simulink model "LDW_mask"  (Simulink 7.8)
settings: Solver=FixedStepDiscrete  StartTime=0.0  StopTime=10.0  FixedStep=1/100  RelTol=1e-3
undefined symbols (not defined in the file or in its folder): High, num_targets, slselsubs
libraries: simulink x35, dspmtrx3 x13, visiontextngfix x9, dspsigops x6, simulink_extras x4, visiontransforms x4, dspstat3 x4, dspswit3 x3, dspadpt3 x3, dspindex x2, visionconversions x2, visionstatistics x2
(part 2 of 3)

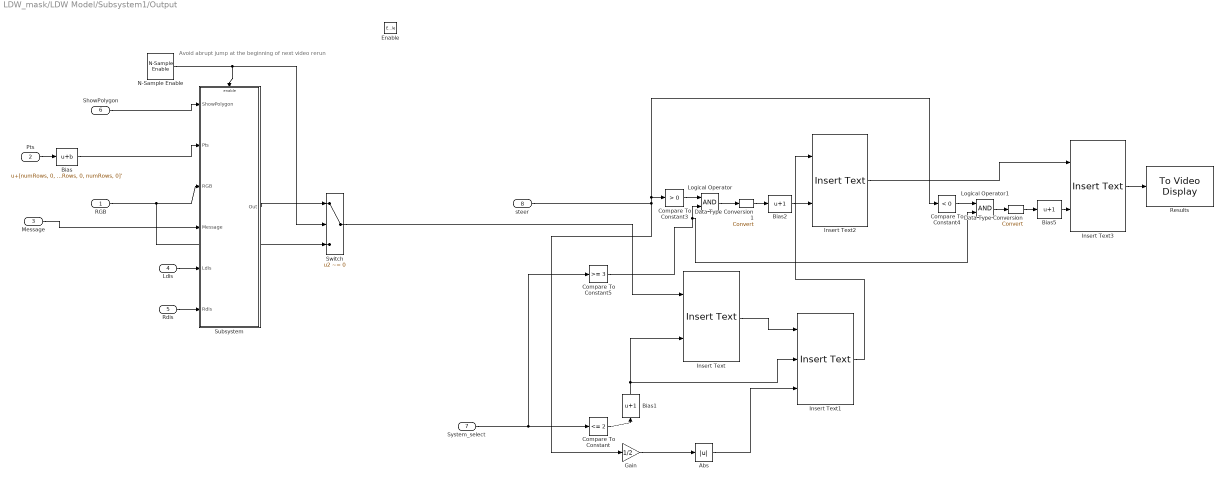
== system LDW_mask/LDW Model/Subsystem1/Output ==
  note: Avoid abrupt jump at the beginning of next video rerun
  RGB : Inport
  Pts : Inport  Port=2
  Message : Inport  Port=3
  Ldis : Inport  Port=4
  Rdis : Inport  Port=5
  ShowPolygon : Inport  Port=6
  System_select : Inport  Port=7
  steer : Inport  Port=8
  Enable : EnablePort
  Abs : Abs
  Bias : Bias  Bias=[numRows, 0, numRows, 0; numRows, 0, numRows, 0]'
  Bias1 : Bias  Bias=1
  Bias2 : Bias  Bias=1
  Bias5 : Bias  Bias=1
  Compare To Constant : simulink/Logic and Bit Operations/Compare To Constant  relop=<=  const=2  OutDataTypeStr=uint8
  Compare To Constant3 : simulink/Logic and Bit Operations/Compare To Constant  relop=>  const=0  OutDataTypeStr=uint8
  Compare To Constant4 : simulink/Logic and Bit Operations/Compare To Constant  relop=<  const=0  OutDataTypeStr=uint8
  Compare To Constant5 : simulink/Logic and Bit Operations/Compare To Constant  relop=>=  const=3  OutDataTypeStr=uint8
  Data Type Conversion : DataTypeConversion
  Data Type Conversion1 : DataTypeConversion
  Gain : Gain  Gain=1/2  OutDataTypeStr=Inherit: Inherit via back propagation
  Insert Text : visiontextngfix/Insert Text  inputType=Obsolete  theText={'Steer:' , ''}  fontFace=LucidaTypewriterBold  dummyVar1=0  blockFontSize=14  antiAliased=on  getTextLocFrom=Specify via dialog  textLoc=[240 10]  getTextColorFrom=Specify via dialog  textColor=[210/255 105/255 30/255]  getTextIntensityFrom=Specify via dialog  textIntensity=0  getTextOpacityFrom=Specify via dialog  textOpacity=1  dummyVar2=0  dummyVar3=0  dummyVar4=0  imagePorts=One multidimensional signal  isInputTransposed=off
  Insert Text1 : visiontextngfix/Insert Text  inputType=Obsolete  theText={[' %6.1f%%'] , ''}  fontFace=LucidaTypewriterBold  dummyVar1=0  blockFontSize=14  antiAliased=on  getTextLocFrom=Specify via dialog  textLoc=[220 25]  getTextColorFrom=Specify via dialog  textColor=[210/255 105/255 30/255]  getTextIntensityFrom=Specify via dialog  textIntensity=0  getTextOpacityFrom=Specify via dialog  textOpacity=1  dummyVar2=0  dummyVar3=0  dummyVar4=0  imagePorts=One multidimensional signal  isInputTransposed=off
  Insert Text2 : visiontextngfix/Insert Text  inputType=Obsolete  theText={'','Left' }  fontFace=LucidaTypewriterBold  dummyVar1=0  blockFontSize=14  antiAliased=on  getTextLocFrom=Specify via dialog  textLoc=[170 10]  getTextColorFrom=Specify via dialog  textColor=[210/255 105/255 30/255]  getTextIntensityFrom=Specify via dialog  textIntensity=0  getTextOpacityFrom=Specify via dialog  textOpacity=1  dummyVar2=0  dummyVar3=0  dummyVar4=0  imagePorts=One multidimensional signal  isInputTransposed=off
  Insert Text3 : visiontextngfix/Insert Text  inputType=Obsolete  theText={'','Right' }  fontFace=LucidaTypewriterBold  dummyVar1=0  blockFontSize=14  antiAliased=on  getTextLocFrom=Specify via dialog  textLoc=[315 10]  getTextColorFrom=Specify via dialog  textColor=[210/255 105/255 30/255]  getTextIntensityFrom=Specify via dialog  textIntensity=0  getTextOpacityFrom=Specify via dialog  textOpacity=1  dummyVar2=0  dummyVar3=0  dummyVar4=0  imagePorts=One multidimensional signal  isInputTransposed=off
  Logical Operator : Logic  AllPortsSameDT=off  OutDataTypeStr=boolean
  Logical Operator1 : Logic  AllPortsSameDT=off  OutDataTypeStr=boolean
  N-Sample Enable : dspswit3/N-Sample Enable  N=8  ActiveLevel=High (1)  reset=off  TriggerType=Non-zero sample  Ts=vfq  DataType=Logical
  Results : visionsinks/To Video Display  inputType=Obsolete  imagePorts=One multidimensional signal  OutputDevice=On-screen video monitor  fullScreen=off  videoWindowX=19  videoWindowY=34  saveWindowSize=off  videoWindowWidth=500  videoWindowHeight=375  dataOrg=Column-major  openAtMdlStart=on  isWindowOpen=on  inputColorFormat=RGB
  Subsystem : Subsystem
  Switch : Switch  Criteria=u2 ~= 0
  wires:
  Pts/1 -> Bias/1
  Message/1 -> Subsystem/4(Message)
  Bias/1 -> Subsystem/2(Pts)
  Subsystem/1(Out) -> Switch/1
  ShowPolygon/1 -> Subsystem/1(ShowPolygon)
  RGB/1 -> Subsystem/3(RGB), Switch/3
  N-Sample Enable/1 -> Subsystem/Enable, Switch/2
  Switch/1 -> Insert Text/1
  Ldis/1 -> Subsystem/5(Ldis)
  Rdis/1 -> Subsystem/6(Rdis)
  System_select/1 -> Compare To Constant/1, Compare To Constant5/1
  Insert Text/1 -> Insert Text1/1
  Compare To Constant/1 -> Bias1/1
  Gain/1 -> Abs/1
  Logical Operator1/1 -> Data Type Conversion/1
  steer/1 -> Compare To Constant4/1, Compare To Constant3/1, Gain/1
  Compare To Constant3/1 -> Logical Operator/1
  Compare To Constant4/1 -> Logical Operator1/1
  Logical Operator/1 -> Data Type Conversion1/1
  Insert Text2/1 -> Insert Text3/1
  Insert Text1/1 -> Insert Text2/1
  Compare To Constant5/1 -> Logical Operator1/2, Logical Operator/2
  Abs/1 -> Insert Text1/3
  Insert Text3/1 -> Results/1
  Data Type Conversion/1 -> Bias5/1
  Bias5/1 -> Insert Text3/2
  Data Type Conversion1/1 -> Bias2/1
  Bias2/1 -> Insert Text2/2
  Bias1/1 -> Insert Text/2, Insert Text1/2

== system LDW_mask/LDW Model/Subsystem1/ind_light ==
  ind_flag : Inport
  ldw_message : Inport  Port=2
  Compare To Constant : simulink/Logic and Bit Operations/Compare To Constant  relop===  const=2  OutDataTypeStr=uint8
  Compare To Constant1 : Logic  AllPortsSameDT=off  OutDataTypeStr=boolean
  Compare To Constant2 : Logic  AllPortsSameDT=off  OutDataTypeStr=boolean
  Compare To Constant3 : Logic  Operator=NOT  AllPortsSameDT=off  OutDataTypeStr=boolean
  Constant : Constant  Value=0
  Constant1 : Constant  Value=0
  Pulse Generator : DiscretePulseGenerator  Period=76  PulseWidth=76/2  SampleTime=Ts_ind
  Pulse Generator1 : DiscretePulseGenerator  Period=76  PulseWidth=76/2  SampleTime=Ts_ind
  Rate Transition : RateTransition  OutPortSampleTimeOpt=Inherit
  Rate Transition1 : RateTransition  OutPortSampleTimeOpt=Inherit
  Switch : Switch  Criteria=u2 > Threshold  Threshold=0.5
  Switch1 : Switch  Criteria=u2 > Threshold  Threshold=0.5
  no : simulink/Logic and Bit Operations/Compare To Constant  relop===  const=0  OutDataTypeStr=uint8
  light_left : Outport
  light_right : Outport  Port=2
  wires:
  Pulse Generator/1 -> Switch/1
  Switch/1 -> light_left/1
  Constant/1 -> Switch/3
  Pulse Generator1/1 -> Switch1/1
  Constant1/1 -> Switch1/3
  Switch1/1 -> light_right/1
  ldw_message/1 -> Compare To Constant/1, no/1
  Compare To Constant/1 -> Compare To Constant2/2
  Compare To Constant2/1 -> Rate Transition1/1
  Compare To Constant1/1 -> Rate Transition/1
  no/1 -> Compare To Constant1/1
  Rate Transition/1 -> Switch1/2
  Rate Transition1/1 -> Switch/2
  ind_flag/1 -> Compare To Constant3/1
  Compare To Constant3/1 -> Compare To Constant2/1, Compare To Constant1/2

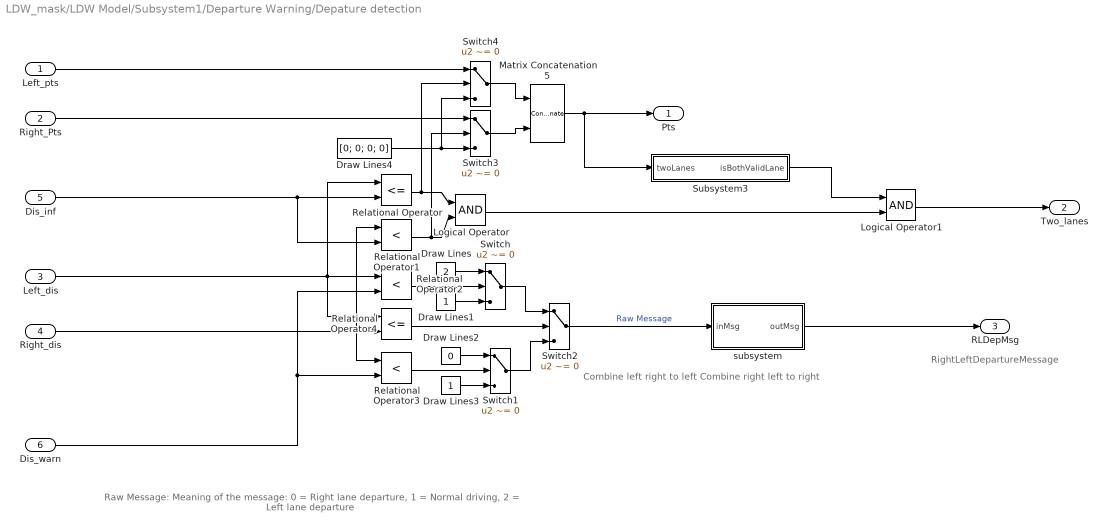
== system LDW_mask/LDW Model/Subsystem1/Departure Warning/Depature detection ==
  note: Raw Message:
      | Meaning of the message: 0 = Right lane departure, 1 = Normal driving, 2 = Left lane departure
  note: RightLeftDepartureMessage
  note: Combine left right to left
      | Combine right left to right
  Left_pts : Inport
  Right_Pts : Inport  Port=2
  Left_dis : Inport  Port=3
  Right_dis : Inport  Port=4
  Dis_inf : Inport  Port=5
  Dis_warn : Inport  Port=6
  Draw Lines : Constant  Value=2  VectorParams1D=off  OutDataTypeStr=int8  SampleTime=cfq
  Draw Lines1 : Constant  VectorParams1D=off  OutDataTypeStr=int8  SampleTime=cfq
  Draw Lines2 : Constant  Value=0  VectorParams1D=off  OutDataTypeStr=int8  SampleTime=cfq
  Draw Lines3 : Constant  VectorParams1D=off  OutDataTypeStr=int8  SampleTime=cfq
  Draw Lines4 : Constant  Value=[0; 0; 0; 0]  VectorParams1D=off  OutDataTypeStr=int32  SampleTime=cfq
  Logical Operator : Logic  AllPortsSameDT=off  OutDataTypeStr=boolean
  Logical Operator1 : Logic  AllPortsSameDT=off  OutDataTypeStr=boolean  SampleTime=cfq
  Matrix Concatenation5 : Concatenate  Mode=Multidimensional array  ConcatenateDimension=2
  Relational Operator : RelationalOperator  Operator=<=  OutDataTypeStr=boolean  ZeroCross=off
  Relational Operator1 : RelationalOperator  Operator=<  OutDataTypeStr=boolean  ZeroCross=off
  Relational Operator2 : RelationalOperator  Operator=<  OutDataTypeStr=boolean  ZeroCross=off
  Relational Operator3 : RelationalOperator  Operator=<  OutDataTypeStr=boolean  ZeroCross=off
  Relational Operator4 : RelationalOperator  Operator=<=  OutDataTypeStr=boolean  ZeroCross=off
  Subsystem3 : Subsystem
  Switch : Switch  Criteria=u2 ~= 0
  Switch1 : Switch  Criteria=u2 ~= 0
  Switch2 : Switch  Criteria=u2 ~= 0
  Switch3 : Switch  Criteria=u2 ~= 0  ZeroCross=off
  Switch4 : Switch  Criteria=u2 ~= 0  ZeroCross=off
  subsystem : Subsystem
  Pts : Outport
  Two_lanes : Outport  Port=2
  RLDepMsg : Outport  Port=3
  wires:
  Relational Operator1/1 -> Logical Operator/2, Switch3/2
  Relational Operator/1 -> Logical Operator/1, Switch4/2
  Switch1/1 -> Switch2/3
  Switch/1 -> Switch2/1
  Relational Operator4/1 -> Switch2/2
  Draw Lines3/1 -> Switch1/3
  Draw Lines2/1 -> Switch1/1
  Draw Lines1/1 -> Switch/3
  Draw Lines/1 -> Switch/1
  Relational Operator3/1 -> Switch1/2
  Relational Operator2/1 -> Switch/2
  Dis_warn/1 -> Relational Operator2/2, Relational Operator3/2
  Left_dis/1 -> Relational Operator2/1, Relational Operator4/1, Relational Operator/1
  Right_dis/1 -> Relational Operator1/1, Relational Operator4/2, Relational Operator3/1
  Dis_inf/1 -> Relational Operator/2, Relational Operator1/2
  Switch3/1 -> Matrix Concatenation5/2
  Switch4/1 -> Matrix Concatenation5/1
  Draw Lines4/1 -> Switch3/3, Switch4/3
  Left_pts/1 -> Switch4/1
  Matrix Concatenation5/1 -> Subsystem3/1(twoLanes), Pts/1
  Right_Pts/1 -> Switch3/1
  Switch2/1 -> subsystem/1(inMsg)  "Raw Message"
  subsystem/1(outMsg) -> RLDepMsg/1
  Subsystem3/1(isBothValidLane) -> Logical Operator1/1
  Logical Operator/1 -> Logical Operator1/2
  Logical Operator1/1 -> Two_lanes/1

== system LDW_mask/LDW Model/Subsystem1/Departure Warning/Depature detection1 ==
  note: Combine left right to left
      | Combine right left to right
  note: RightLeftDepartureMessage
  Left_dis : Inport
  Right_dis : Inport  Port=2
  Dis_LDW_warn : Inport  Port=3
  Enable : EnablePort
  Draw Lines : Constant  Value=2  VectorParams1D=off  OutDataTypeStr=int8  SampleTime=cfq
  Draw Lines1 : Constant  VectorParams1D=off  OutDataTypeStr=int8  SampleTime=cfq
  Draw Lines2 : Constant  Value=0  VectorParams1D=off  OutDataTypeStr=int8  SampleTime=cfq
  Draw Lines3 : Constant  VectorParams1D=off  OutDataTypeStr=int8  SampleTime=cfq
  Relational Operator2 : RelationalOperator  Operator=<  OutDataTypeStr=boolean  ZeroCross=off
  Relational Operator3 : RelationalOperator  Operator=<  OutDataTypeStr=boolean  ZeroCross=off
  Relational Operator4 : RelationalOperator  Operator=<=  OutDataTypeStr=boolean  ZeroCross=off
  Switch : Switch  Criteria=u2 ~= 0
  Switch1 : Switch  Criteria=u2 ~= 0
  Switch2 : Switch  Criteria=u2 ~= 0
  subsystem : Subsystem
  LDW_Asist_flag : Outport
  wires:
  subsystem/1(outMsg) -> LDW_Asist_flag/1
  Switch2/1 -> subsystem/1(inMsg)  "Raw Massage"
  Right_dis/1 -> Relational Operator3/1, Relational Operator4/2
  Left_dis/1 -> Relational Operator4/1, Relational Operator2/1
  Dis_LDW_warn/1 -> Relational Operator3/2, Relational Operator2/2
  Relational Operator2/1 -> Switch/2
  Relational Operator3/1 -> Switch1/2
  Draw Lines/1 -> Switch/1
  Draw Lines1/1 -> Switch/3
  Draw Lines2/1 -> Switch1/1
  Draw Lines3/1 -> Switch1/3
  Relational Operator4/1 -> Switch2/2
  Switch/1 -> Switch2/1
  Switch1/1 -> Switch2/3

== system LDW_mask/LDW Model/Subsystem1/Departure Warning/Find the left and  right lanes from the depository ==
  note: Left and right lanes are identified by their intersection positions with the bottom image boundary.
      | The intersection point of the left lane is to the left of the image bottom boundary center,
      | and is the one closest to the center. By the same way, but to the right, the right lane is defined.
  Count : Inport
  Pts : Inport  Port=2
  Half_width : Inport  Port=3
  Dis_inf : Inport  Port=4
  Compare To Constant2 : simulink/Logic and Bit Operations/Compare To Constant  relop=>=  const=frameFound  OutDataTypeStr=boolean  ZeroCross=off
  For Iterator : ForIterator  ResetStates=reset  IterationLimit=maxLaneNum
  Search for the left and right lanes : Subsystem
  select rho1 : Selector  NumberOfDimensions=2  InputPortWidth=maxLaneNum  IndexOptions=Select all,Index vector (port)  Indices=-1,-1  OutputSizes=1
  select rho5 : Selector  NumberOfDimensions=2  InputPortWidth=maxLaneNum  IndexOptions=Select all,Index vector (port)  Indices=-1,-1  OutputSizes=1
  Left_pts : Outport
  Left_dis : Outport  Port=2
  wires:
  Pts/1 -> select rho5/1
  select rho1/1 -> Compare To Constant2/1
  Half_width/1 -> Search for the left and right lanes/3(Half_width)
  select rho5/1 -> Search for the left and right lanes/2(Pts)
  Compare To Constant2/1 -> Search for the left and right lanes/1(Enable)
  Search for the left and right lanes/1(Left_pts) -> Left_pts/1
  Search for the left and right lanes/2(Left_dis) -> Left_dis/1
  For Iterator/1 -> select rho5/2, select rho1/2
  Count/1 -> select rho1/1
  Dis_inf/1 -> Search for the left and right lanes/4(Dis_inf)

== system LDW_mask/LDW Model/Subsystem1/Departure Warning/Find the left and  right lanes from the depository1 ==
  note: Left and right lanes are identified by their intersection positions with the bottom image boundary.
      | The intersection point of the left lane is to the left of the image bottom boundary center,
      | and is the one closest to the center. By the same way, but to the right, the right lane is defined.
  Count : Inport
  Pts : Inport  Port=2
  Half_width : Inport  Port=3
  Dis_inf : Inport  Port=4
  Compare To Constant2 : simulink/Logic and Bit Operations/Compare To Constant  relop=>=  const=frameFound  OutDataTypeStr=boolean  ZeroCross=off
  For Iterator : ForIterator  ResetStates=reset  IterationLimit=maxLaneNum
  Search for the left and right lanes : Subsystem
  select rho1 : Selector  NumberOfDimensions=2  InputPortWidth=maxLaneNum  IndexOptions=Select all,Index vector (port)  Indices=-1,-1  OutputSizes=1
  select rho5 : Selector  NumberOfDimensions=2  InputPortWidth=maxLaneNum  IndexOptions=Select all,Index vector (port)  Indices=-1,-1  OutputSizes=1
  Right_pts : Outport
  Right_dis : Outport  Port=2
  wires:
  Dis_inf/1 -> Search for the left and right lanes/4(Dis_inf)
  Count/1 -> select rho1/1
  For Iterator/1 -> select rho1/2, select rho5/2
  Search for the left and right lanes/2(Left_dis) -> Right_dis/1
  Search for the left and right lanes/1(Left_pts) -> Right_pts/1
  Compare To Constant2/1 -> Search for the left and right lanes/1(Enable)
  select rho5/1 -> Search for the left and right lanes/2(Pts)
  Half_width/1 -> Search for the left and right lanes/3(Half_width)
  select rho1/1 -> Compare To Constant2/1
  Pts/1 -> select rho5/1

== system LDW_mask/LDW Model/Subsystem1/Departure Warning/Subsystem ==
  left_pts : Inport
  right_pts : Inport  Port=2
  left_dist : Inport  Port=3
  right_dist : Inport  Port=4
  MATLAB Function3 : MATLAB Function  TreatAsAtomicUnit=on
  Multiport Switch{,1..3} (4 alike) : MultiPortSwitch  Inputs=2  zeroidx=off  SampleTime=cfq
  Unit Delay{,1..3} (4 alike) : UnitDelay  SampleTime=-1
  left_points : Outport
  right_points : Outport  Port=2
  left_distance : Outport  Port=3
  right_distance : Outport  Port=4
  wires:
  left_pts/1 -> MATLAB Function3/1(L_pts), Multiport Switch/2
  right_pts/1 -> MATLAB Function3/2(R_pts), Multiport Switch1/2
  Multiport Switch/1 -> Unit Delay/1, left_points/1
  Multiport Switch1/1 -> Unit Delay1/1, right_points/1
  Multiport Switch2/1 -> Unit Delay2/1, left_distance/1
  Unit Delay/1 -> Multiport Switch/3
  Unit Delay1/1 -> Multiport Switch1/3
  Unit Delay2/1 -> Multiport Switch2/3
  Unit Delay3/1 -> Multiport Switch3/3
  left_dist/1 -> Multiport Switch2/2
  right_dist/1 -> Multiport Switch3/2
  Multiport Switch3/1 -> right_distance/1, Unit Delay3/1
  MATLAB Function3/1(swch) -> Multiport Switch/1, Multiport Switch1/1, Multiport Switch2/1, Multiport Switch3/1

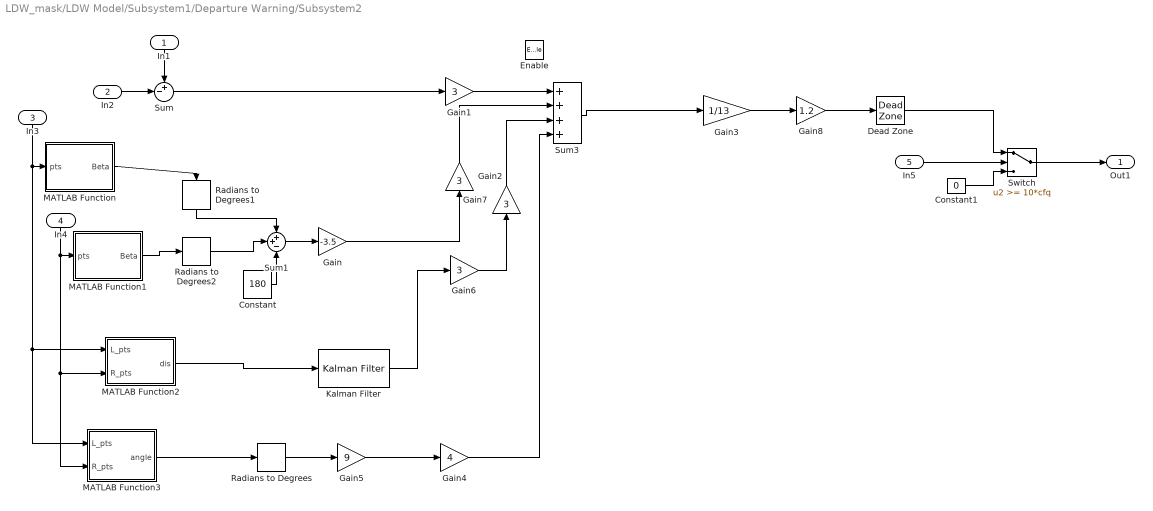
== system LDW_mask/LDW Model/Subsystem1/Departure Warning/Subsystem2 ==
  In1 : Inport
  In2 : Inport  Port=2
  In3 : Inport  Port=3
  In4 : Inport  Port=4
  In5 : Inport  Port=5
  Enable : EnablePort
  Constant : Constant  Value=180  SampleTime=cfq
  Constant1 : Constant  Value=0  SampleTime=cfq
  Dead Zone : DeadZone  LowerValue=-15  UpperValue=15  SaturateOnIntegerOverflow=on
  Gain : Gain  Gain=-3.5
  Gain1 : Gain  Gain=3  OutDataTypeStr=int32
  Gain2 : Gain  Gain=3
  Gain3 : Gain  Gain=1/13  OutDataTypeStr=int32
  Gain4 : Gain  Gain=4
  Gain5 : Gain  Gain=9
  Gain6 : Gain  Gain=3
  Gain7 : Gain  Gain=3
  Gain8 : Gain  Gain=1.2  OutDataTypeStr=int32
  Kalman Filter : dspadpt3/Kalman Filter  num_targets=1  sourceEnable=Always  isReset=on  X=zeros([1, 1])  P=10*eye(1)  A=1  sourceMeasure=Specify via Dialog  H=1  Q=0.05*eye(1)  R=5  isOutputEstMeasure=on  isOutputEstState=off  isOutputEstError=off  isOutputPrdMeasure=off  isOutputPrdState=off  isOutputPrdError=off
  MATLAB Function : MATLAB Function  TreatAsAtomicUnit=on
  MATLAB Function1 : MATLAB Function  TreatAsAtomicUnit=on
  MATLAB Function2 : MATLAB Function  TreatAsAtomicUnit=on
  MATLAB Function3 : MATLAB Function  TreatAsAtomicUnit=on
  Radians to Degrees : simulink_extras/Transformations/Radians to Degrees
  Radians to Degrees1 : simulink_extras/Transformations/Radians to Degrees
  Radians to Degrees2 : simulink_extras/Transformations/Radians to Degrees
  Sum : Sum  Inputs=+-|  AccumDataTypeStr=int32  OutDataTypeStr=int32
  Sum1 : Sum  Inputs=++-  AccumDataTypeStr=double  OutDataTypeStr=double
  Sum3 : Sum  Inputs=++++  AccumDataTypeStr=int32  OutDataTypeStr=single
  Switch : Switch  Threshold=10*cfq  SampleTime=cfq
  Out1 : Outport
  wires:
  Radians to Degrees/1 -> Gain5/1
  Gain5/1 -> Gain4/1
  Gain4/1 -> Sum3/4
  MATLAB Function3/1(angle) -> Radians to Degrees/1
  Dead Zone/1 -> Switch/1
  In5/1 -> Switch/2
  Switch/1 -> Out1/1
  Constant1/1 -> Switch/3
  Gain8/1 -> Dead Zone/1
  In4/1 -> MATLAB Function2/2(R_pts), MATLAB Function3/2(R_pts), MATLAB Function1/1(pts)
  In3/1 -> MATLAB Function2/1(L_pts), MATLAB Function3/1(L_pts), MATLAB Function/1(pts)
  In2/1 -> Sum/2
  In1/1 -> Sum/1
  Gain7/1 -> Sum3/3
  Gain6/1 -> Gain7/1
  Gain3/1 -> Gain8/1
  Gain2/1 -> Sum3/2
  Gain1/1 -> Sum3/1
  Sum3/1 -> Gain3/1
  Kalman Filter/1 -> Gain6/1
  Gain/1 -> Gain2/1
  Radians to Degrees2/1 -> Sum1/2
  Radians to Degrees1/1 -> Sum1/1
  Constant/1 -> Sum1/3
  MATLAB Function2/1(dis) -> Kalman Filter/1
  Sum1/1 -> Gain/1
  MATLAB Function1/1(Beta) -> Radians to Degrees2/1
  MATLAB Function/1(Beta) -> Radians to Degrees1/1
  Sum/1 -> Gain1/1

== system LDW_mask/LDW Model/Subsystem1/Departure Warning/Subsystem3 ==
  left_pts : Inport
  right_pts : Inport  Port=2
  left_dist : Inport  Port=3
  right_dist : Inport  Port=4
  Bias : Bias  Bias=[0, imgSize(2), 0, imgSize(2)]'
  Embedded MATLAB Function : MATLAB Function  TreatAsAtomicUnit=on
  Embedded MATLAB Function1 : MATLAB Function  TreatAsAtomicUnit=on
  Gain : Gain  Gain=[1, -1, 1, -1]'  OutDataTypeStr=Inherit: Inherit via back propagation
  Unit Delay{,1..3} (4 alike) : UnitDelay  SampleTime=cfq
  left_points : Outport
  right_points : Outport  Port=2
  left_distance : Outport  Port=3
  right_distance : Outport  Port=4
  wires:
  left_pts/1 -> Embedded MATLAB Function/1(pts_in)
  left_dist/1 -> Embedded MATLAB Function/2(dist_in)
  Embedded MATLAB Function/1(pts_out) -> Unit Delay1/1, left_points/1
  Embedded MATLAB Function/2(dist_out) -> Unit Delay/1, left_distance/1
  Unit Delay1/1 -> Embedded MATLAB Function/3(pts_prev)
  right_pts/1 -> Embedded MATLAB Function1/1(pts_in)
  right_dist/1 -> Embedded MATLAB Function1/2(dist_in)
  Embedded MATLAB Function1/1(pts_out) -> Unit Delay3/1, Gain/1
  Embedded MATLAB Function1/2(dist_out) -> Unit Delay2/1, right_distance/1
  Unit Delay2/1 -> Embedded MATLAB Function1/4(dist_prev)
  Unit Delay3/1 -> Embedded MATLAB Function1/3(pts_prev)
  Gain/1 -> Bias/1
  Bias/1 -> right_points/1
  Unit Delay/1 -> Embedded MATLAB Function/4(dist_prev)

== system LDW_mask/LDW Model/Subsystem1/Lane Detection/Overwrite ==
  note: Wipe out Hamtrix with
      | theta >=  78deg
  note: Wipe out Hamtrix with
      | theta <  -78deg
  In : Inport
  Overwrite Values : dspmtrx3/Overwrite Values  OverWriteDiag=Submatrix  valFrom2ndIP=Specify via dialog  ConstValue=0  RowSpan=All rows  RowStartMode=First  RowStartIndex=1  RowEndMode=Last  RowEndIndex=1  ColSpan=Range of columns  ColStartMode=First  ColStartIndex=1  ColEndMode=Index  ColEndIndex=12  DiagSpan=Range of elements  DiagStartMode=Index  DiagStartIndex=2  DiagEndMode=Index  DiagEndIndex=4
  Overwrite Values1 : dspmtrx3/Overwrite Values  OverWriteDiag=Submatrix  valFrom2ndIP=Specify via dialog  ConstValue=0  RowSpan=All rows  RowStartMode=First  RowStartIndex=1  RowEndMode=Last  RowEndIndex=1  ColSpan=Range of columns  ColStartMode=Offset from last  ColStartIndex=12  ColEndMode=Last  ColEndIndex=15  DiagSpan=Range of elements  DiagStartMode=Index  DiagStartIndex=2  DiagEndMode=Index  DiagEndIndex=4
  Out : Outport
  wires:
  Overwrite Values/1 -> Overwrite Values1/1
  In/1 -> Overwrite Values/1
  Overwrite Values1/1 -> Out/1

== system LDW_mask/LDW Model/Subsystem1/Lane Detection/Overwrite1 ==
  note: Wipe out Hamtrix with
      | theta <  -78deg
  note: Wipe out Hamtrix with
      | theta >=  78deg
  In : Inport
  Overwrite Values : dspmtrx3/Overwrite Values  OverWriteDiag=Submatrix  valFrom2ndIP=Specify via dialog  ConstValue=0  RowSpan=All rows  RowStartMode=First  RowStartIndex=1  RowEndMode=Last  RowEndIndex=1  ColSpan=Range of columns  ColStartMode=First  ColStartIndex=1  ColEndMode=Index  ColEndIndex=12  DiagSpan=Range of elements  DiagStartMode=Index  DiagStartIndex=2  DiagEndMode=Index  DiagEndIndex=4
  Overwrite Values1 : dspmtrx3/Overwrite Values  OverWriteDiag=Submatrix  valFrom2ndIP=Specify via dialog  ConstValue=0  RowSpan=All rows  RowStartMode=First  RowStartIndex=1  RowEndMode=Last  RowEndIndex=1  ColSpan=Range of columns  ColStartMode=Offset from last  ColStartIndex=12  ColEndMode=Last  ColEndIndex=15  DiagSpan=Range of elements  DiagStartMode=Index  DiagStartIndex=2  DiagEndMode=Index  DiagEndIndex=4
  Out : Outport
  wires:
  Overwrite Values1/1 -> Out/1
  In/1 -> Overwrite Values/1
  Overwrite Values/1 -> Overwrite Values1/1

== system LDW_mask/LDW Model/Subsystem1/Lane Detection/Peak detection ==
  note: Detect lines in the image by finding the peaks in the Hough transform matrix
  Hough : Inport
  Theta_list : Inport  Port=2
  Rho_list : Inport  Port=3
  Enable signal generator : Subsystem  TreatAsAtomicUnit=on
  Find Local Maxima1 : visionstatistics/Find Local Maxima  num_peaks=expLaneNum  nhood_size=neighborhood  src_thresh=Obsolete9b  src_thresh_inuse=Specify via dialog  threshold=1  inputIsHough=on  dt_peak=uint16  isOutVarDim=off  dt_count=uint32
  Matrix Concatenation3 : Concatenate  Mode=Multidimensional array
  Probe : Probe  ProbeWidth=off  ProbeSampleTime=off  ProbeComplexSignal=off  ProbeSignalDimensions=on
  Selector : Selector  NumberOfDimensions=2  InputPortWidth=3  IndexOptions=Index vector (dialog),Index vector (dialog)  Indices=1,2  OutputSizes=1,1
  Selector rho : Selector  NumberOfDimensions=2  IndexMode=Zero-based  InputPortWidth=3  IndexOptions=Select all,Index vector (port)  Indices=1,2  OutputSizes=1,1
  Selector theta : Selector  NumberOfDimensions=2  IndexMode=Zero-based  InputPortWidth=3  IndexOptions=Select all,Index vector (port)  Indices=1,2  OutputSizes=1,1
  Selector1 : Selector  NumberOfDimensions=2  InputPortWidth=3  IndexOptions=Select all,Index vector (dialog)  Indices=[2 1],[2 1]  OutputSizes=1,1
  Terminator : Terminator
  Transpose : dspmtrx3/Transpose  Hermitian=off  overflowFlag=off
  Zero-Order Hold1 : ZeroOrderHold  SampleTime=-1
  Zero-Order Hold2 : ZeroOrderHold  SampleTime=-1
  select rho : Selector  NumberOfDimensions=2  InputPortWidth=3  IndexOptions=Index vector (dialog),Select all  Indices=1,-1  OutputSizes=1
  select rho3 : Selector  NumberOfDimensions=2  InputPortWidth=3  IndexOptions=Index vector (dialog),Select all  Indices=2,-1  OutputSizes=1
  Line : Outport
  Enable : Outport  Port=2
  wires:
  Hough/1 -> Find Local Maxima1/1
  Enable signal generator/1(Enable) -> Enable/1
  Matrix Concatenation3/1 -> Line/1
  Selector theta/1 -> Matrix Concatenation3/2
  Selector rho/1 -> Matrix Concatenation3/1
  Zero-Order Hold1/1 -> Selector theta/1
  select rho3/1 -> Selector theta/2
  Theta_list/1 -> Zero-Order Hold1/1
  Zero-Order Hold2/1 -> Selector rho/1
  Transpose/1 -> select rho/1, select rho3/1, Probe/1
  select rho/1 -> Selector rho/2
  Rho_list/1 -> Zero-Order Hold2/1
  Probe/1 -> Selector/1
  Selector/1 -> Enable signal generator/1(Num)
  Find Local Maxima1/2 -> Terminator/1
  Selector1/1 -> Transpose/1
  Find Local Maxima1/1 -> Selector1/1

== system LDW_mask/LDW Model/Subsystem1/Lane Detection/Peak detection1 ==
  note: Detect lines in the image by finding the peaks in the Hough transform matrix
  Hough : Inport
  Theta_list : Inport  Port=2
  Rho_list : Inport  Port=3
  Enable signal generator : Subsystem  TreatAsAtomicUnit=on
  Find Local Maxima1 : visionstatistics/Find Local Maxima  num_peaks=expLaneNum  nhood_size=neighborhood  src_thresh=Obsolete9b  src_thresh_inuse=Specify via dialog  threshold=1  inputIsHough=on  dt_peak=uint16  isOutVarDim=off  dt_count=uint32
  Matrix Concatenation3 : Concatenate  Mode=Multidimensional array
  Probe : Probe  ProbeWidth=off  ProbeSampleTime=off  ProbeComplexSignal=off  ProbeSignalDimensions=on
  Selector : Selector  NumberOfDimensions=2  InputPortWidth=3  IndexOptions=Index vector (dialog),Index vector (dialog)  Indices=1,2  OutputSizes=1,1
  Selector rho : Selector  NumberOfDimensions=2  IndexMode=Zero-based  InputPortWidth=3  IndexOptions=Select all,Index vector (port)  Indices=1,2  OutputSizes=1,1
  Selector theta : Selector  NumberOfDimensions=2  IndexMode=Zero-based  InputPortWidth=3  IndexOptions=Select all,Index vector (port)  Indices=1,2  OutputSizes=1,1
  Selector1 : Selector  NumberOfDimensions=2  InputPortWidth=3  IndexOptions=Select all,Index vector (dialog)  Indices=[2 1],[2 1]  OutputSizes=1,1
  Terminator : Terminator
  Transpose : dspmtrx3/Transpose  Hermitian=off  overflowFlag=off
  Zero-Order Hold1 : ZeroOrderHold  SampleTime=-1
  Zero-Order Hold2 : ZeroOrderHold  SampleTime=-1
  select rho : Selector  NumberOfDimensions=2  InputPortWidth=3  IndexOptions=Index vector (dialog),Select all  Indices=1,-1  OutputSizes=1
  select rho3 : Selector  NumberOfDimensions=2  InputPortWidth=3  IndexOptions=Index vector (dialog),Select all  Indices=2,-1  OutputSizes=1
  Line : Outport
  Enable : Outport  Port=2
  wires:
  Selector/1 -> Enable signal generator/1(Num)
  Probe/1 -> Selector/1
  Rho_list/1 -> Zero-Order Hold2/1
  select rho/1 -> Selector rho/2
  Transpose/1 -> Probe/1, select rho3/1, select rho/1
  Zero-Order Hold2/1 -> Selector rho/1
  Theta_list/1 -> Zero-Order Hold1/1
  select rho3/1 -> Selector theta/2
  Zero-Order Hold1/1 -> Selector theta/1
  Selector rho/1 -> Matrix Concatenation3/1
  Selector theta/1 -> Matrix Concatenation3/2
  Matrix Concatenation3/1 -> Line/1
  Enable signal generator/1(Enable) -> Enable/1
  Hough/1 -> Find Local Maxima1/1
  Find Local Maxima1/2 -> Terminator/1
  Find Local Maxima1/1 -> Selector1/1
  Selector1/1 -> Transpose/1

== system LDW_mask/LDW Model/Subsystem1/Lane Detection/Subsystem ==
  In1 : Inport
  Enable : EnablePort
  Filtered : visionsinks/To Video Display  inputType=Obsolete  imagePorts=One multidimensional signal  OutputDevice=On-screen video monitor  fullScreen=off  videoWindowX=550  videoWindowY=830  saveWindowSize=off  videoWindowWidth=500  videoWindowHeight=110  dataOrg=Column-major  openAtMdlStart=on  isWindowOpen=on  inputColorFormat=RGB
  wires:
  In1/1 -> Filtered/1

== system LDW_mask/LDW Model/Subsystem1/Lane Tracking/Matching ==
  Line : Inport
  Enable : Inport  Port=2
  Rep_ref : Inport  Port=3
  Count_ref : Inport  Port=4
  Calculate the distances between  the lines found in the current  frame and those in the respository : Subsystem  TreatAsAtomicUnit=on
  Find the best  matches between the current  lines and those in the repository : Subsystem  TreatAsAtomicUnit=on
  Update the repository : Subsystem  TreatAsAtomicUnit=on
  Repository : Outport
  Count : Outport  Port=2
  wires:
  Find the best  matches between the current  lines and those in the repository/2(Match_dis) -> Update the repository/4(Match_dis)
  Calculate the distances between  the lines found in the current  frame and those in the respository/1(Dis) -> Find the best  matches between the current  lines and those in the repository/1(Dis)
  Enable/1 -> Calculate the distances between  the lines found in the current  frame and those in the respository/4(Enable)
  Rep_ref/1 -> Calculate the distances between  the lines found in the current  frame and those in the respository/2(Rep_ref), Update the repository/1(Rep_ref)
  Line/1 -> Calculate the distances between  the lines found in the current  frame and those in the respository/3(Line), Update the repository/5(Line)
  Find the best  matches between the current  lines and those in the repository/1(Match_list) -> Update the repository/3(Match_list)
  Update the repository/1(Repository) -> Repository/1
  Update the repository/2(Count) -> Count/1
  Count_ref/1 -> Update the repository/2(Count_ref), Calculate the distances between  the lines found in the current  frame and those in the respository/1(Count)

== system LDW_mask/LDW Model/Subsystem1/Lane Tracking/Update ==
  note: For each element (column), Out equals to New if Enable is true; or equals to Old otherwise.
  Old : Inport
  New : Inport  Port=2
  Update : Inport  Port=3
  Assignment : Assignment  NumberOfDimensions=2  IndexOptions=Assign all,Index vector (port)  Indices=-1,-1  OutputSizes=1,1
  For Iterator : ForIterator  ResetStates=reset  IterationLimit=maxLaneNum
  Selector : Selector  InputPortWidth=maxLaneNum  IndexOptions=Index vector (port)  Indices=[1 3]  OutputSizes=1
  Selector1 : Selector  NumberOfDimensions=2  InputPortWidth=maxLaneNum  IndexOptions=Select all,Index vector (port)  Indices=-1,1  OutputSizes=1
  Selector2 : Selector  NumberOfDimensions=2  InputPortWidth=maxLaneNum  IndexOptions=Select all,Index vector (port)  Indices=-1,1  OutputSizes=1
  Switch1 : Switch  Criteria=u2 ~= 0
  Out : Outport
  wires:
  Switch1/1 -> Assignment/2
  Selector/1 -> Switch1/2
  Selector2/1 -> Switch1/3
  Selector1/1 -> Switch1/1
  New/1 -> Assignment/1, Selector1/1
  Old/1 -> Selector2/1
  Assignment/1 -> Out/1
  Update/1 -> Selector/1
  For Iterator/1 -> Assignment/3, Selector1/2, Selector2/2, Selector/2

== system LDW_mask/LDW Model/Subsystem1/Lane Tracking1/Matching ==
  Line : Inport
  Enable : Inport  Port=2
  Rep_ref : Inport  Port=3
  Count_ref : Inport  Port=4
  Calculate the distances between  the lines found in the current  frame and those in the respository : Subsystem  TreatAsAtomicUnit=on
  Find the best  matches between the current  lines and those in the repository : Subsystem  TreatAsAtomicUnit=on
  Update the repository : Subsystem  TreatAsAtomicUnit=on
  Repository : Outport
  Count : Outport  Port=2
  wires:
  Count_ref/1 -> Calculate the distances between  the lines found in the current  frame and those in the respository/1(Count), Update the repository/2(Count_ref)
  Update the repository/2(Count) -> Count/1
  Update the repository/1(Repository) -> Repository/1
  Find the best  matches between the current  lines and those in the repository/1(Match_list) -> Update the repository/3(Match_list)
  Line/1 -> Calculate the distances between  the lines found in the current  frame and those in the respository/3(Line), Update the repository/5(Line)
  Rep_ref/1 -> Calculate the distances between  the lines found in the current  frame and those in the respository/2(Rep_ref), Update the repository/1(Rep_ref)
  Enable/1 -> Calculate the distances between  the lines found in the current  frame and those in the respository/4(Enable)
  Calculate the distances between  the lines found in the current  frame and those in the respository/1(Dis) -> Find the best  matches between the current  lines and those in the repository/1(Dis)
  Find the best  matches between the current  lines and those in the repository/2(Match_dis) -> Update the repository/4(Match_dis)

== system LDW_mask/LDW Model/Subsystem1/Lane Tracking1/Update ==
  note: For each element (column), Out equals to New if Enable is true; or equals to Old otherwise.
  Old : Inport
  New : Inport  Port=2
  Update : Inport  Port=3
  Assignment : Assignment  NumberOfDimensions=2  IndexOptions=Assign all,Index vector (port)  Indices=-1,-1  OutputSizes=1,1
  For Iterator : ForIterator  ResetStates=reset  IterationLimit=maxLaneNum
  Selector : Selector  InputPortWidth=maxLaneNum  IndexOptions=Index vector (port)  Indices=[1 3]  OutputSizes=1
  Selector1 : Selector  NumberOfDimensions=2  InputPortWidth=maxLaneNum  IndexOptions=Select all,Index vector (port)  Indices=-1,1  OutputSizes=1
  Selector2 : Selector  NumberOfDimensions=2  InputPortWidth=maxLaneNum  IndexOptions=Select all,Index vector (port)  Indices=-1,1  OutputSizes=1
  Switch1 : Switch  Criteria=u2 ~= 0
  Out : Outport
  wires:
  For Iterator/1 -> Selector/2, Selector2/2, Selector1/2, Assignment/3
  Update/1 -> Selector/1
  Assignment/1 -> Out/1
  Old/1 -> Selector2/1
  New/1 -> Selector1/1, Assignment/1
  Selector1/1 -> Switch1/1
  Selector2/1 -> Switch1/3
  Selector/1 -> Switch1/2
  Switch1/1 -> Assignment/2

== system LDW_mask/LDW Model/Subsystem1/Output/Subsystem ==
  note: Message:
      | 0 = Right lane departure, 1 = Normal driving, 2 = Left lane departure
  ShowPolygon : Inport
  Pts : Inport  Port=2
  RGB : Inport  Port=3
  Message : Inport  Port=4
  Ldis : Inport  Port=5
  Rdis : Inport  Port=6
  Enable : EnablePort  PropagateVarSize=During execution
  Bias : Bias  Bias=1
  Draw  Polygon : Subsystem  TreatAsAtomicUnit=on
  Draw Color and Marker Type : Subsystem
  DrawShapes : visiontextngfix/Draw Shapes  shape=Lines  fill=on  fillClrSource=Specify via dialog  display=User-specified value  intensity=200  color=[1 1 0; 1 0 1]  opacity=0.6  viewport=Entire image  antialiasing=on  inType=Obsolete  imagePorts=One multidimensional signal  prodOutputMode=Binary point scaling  prodOutputWordLength=32  prodOutputFracLength=14  memoryMode=Specify word length  memoryWordLength=16  memoryFracLength=14  roundingMode=Floor  overflowMode=off
  Insert Text1 : visiontextngfix/Insert Text  inputType=Obsolete  theText="{sprintf('                    Right\\n                    Departure'),'',sprintf(' Left\\n Departure')}"  fontFace=LucidaTypewriterBold  dummyVar1=0  blockFontSize=20  antiAliased=on  getTextLocFrom=Specify via dialog  textLoc=[2 170]  getTextColorFrom=Input port  textColor=[1 1 1]  getTextIntensityFrom=Specify via dialog  textIntensity=0  getTextOpacityFrom=Specify via dialog  textOpacity=1  dummyVar2=0  dummyVar3=0  dummyVar4=0  imagePorts=One multidimensional signal  isInputTransposed=off
  Selector2 : Selector  NumberOfDimensions=2  InputPortWidth=3  IndexOptions=Index vector (dialog),Select all  Indices=[2 1 4 3],1  OutputSizes=1,1
  Signal From Workspace : dspsrcs4/Signal From Workspace  X=single([1 0 0;1 0 0; 0 0 0;0 0 0])  Ts=vfq  nsamps=1  OutputAfterFinalValue=Cyclic repetition  ignoreOrWarnInputAndFrameLengths=off
  Switch : Switch  Criteria=u2 ~= 0
  Transpose1 : dspmtrx3/Transpose  Hermitian=off  overflowFlag=off
  Out : Outport
  wires:
  DrawShapes/1 -> Insert Text1/1
  Switch/1 -> DrawShapes/1
  Draw  Polygon/1(RGBout) -> Switch/1
  Signal From Workspace/1 -> Insert Text1/3
  ShowPolygon/1 -> Switch/2, Draw  Polygon/Enable
  RGB/1 -> Draw  Polygon/2(RGB), Switch/3
  Insert Text1/1 -> Draw Color and Marker Type/1(Image)
  Pts/1 -> Selector2/1, Draw  Polygon/1(inPts)
  Message/1 -> Bias/1
  Ldis/1 -> Draw Color and Marker Type/2(Ldis)
  Rdis/1 -> Draw Color and Marker Type/3(Rdis)
  Draw Color and Marker Type/1(Out) -> Out/1
  Selector2/1 -> Transpose1/1
  Transpose1/1 -> DrawShapes/2
  Bias/1 -> Insert Text1/2

== system LDW_mask/LDW Model/Subsystem1/Departure Warning/Depature detection/Subsystem3 ==
  note: c2 C2
  note: c1 C1
  note: r2 R2
  note: r1 R1
  note: Excludes lane [r1 c1 r2 c2]' if:
      | (1) r1 <0
      | (2) abs(r1-c1)+abs(r2-c2) <10
  note: r1
      | r2
      | c1
      | c2
  note: R1
      | R2
      | C1
      | C2
  twoLanes : Inport
  Abs : Abs
  Abs1 : Abs
  Add : Sum  Inputs=+-
  Add1 : Sum  Inputs=+-
  Add2 : Sum
  Compare To Constant1 : simulink/Logic and Bit Operations/Compare To Constant  relop=>=  const=10  OutDataTypeStr=boolean  ZeroCross=off
  Compare To Constant10 : simulink/Logic and Bit Operations/Compare To Constant  relop=>=  const=0  OutDataTypeStr=boolean  ZeroCross=off
  Logical Operator : Logic  AllPortsSameDT=off  OutDataTypeStr=boolean
  Logical Operator7 : Logic  Inputs=3  AllPortsSameDT=off  OutDataTypeStr=boolean
  Logical Operator8 : Logic  Operator=OR  AllPortsSameDT=off  OutDataTypeStr=boolean
  Multiport Selector : dspindex/Multiport Selector  rowsOrCols=Rows  idxCellArray={1,3,2,4}  idxErrMode=Generate Error
  Multiport Selector1 : dspindex/Multiport Selector  rowsOrCols=Columns  idxCellArray={1,2}  idxErrMode=Generate Error
  Relational Operator : RelationalOperator  Operator=~=  OutDataTypeStr=boolean
  Relational Operator1 : RelationalOperator  Operator=~=  OutDataTypeStr=boolean
  isBothValidLane : Outport
  wires:
  Multiport Selector/2 -> Add/2, Relational Operator/2
  Compare To Constant1/1 -> Logical Operator7/3
  Add2/1 -> Compare To Constant1/1
  Abs1/1 -> Add2/2
  Abs/1 -> Add2/1
  Add/1 -> Abs/1
  Add1/1 -> Abs1/1
  Logical Operator8/1 -> Logical Operator7/2
  Relational Operator1/1 -> Logical Operator8/2
  Relational Operator/1 -> Logical Operator8/1
  Multiport Selector/4 -> Add1/2, Relational Operator1/2
  Multiport Selector/3 -> Add1/1, Relational Operator1/1
  Multiport Selector/1 -> Add/1, Compare To Constant10/1, Relational Operator/1
  twoLanes/1 -> Multiport Selector/1
  Compare To Constant10/1 -> Logical Operator7/1
  Logical Operator7/1 -> Multiport Selector1/1
  Multiport Selector1/1 -> Logical Operator/1
  Multiport Selector1/2 -> Logical Operator/2
  Logical Operator/1 -> isBothValidLane/1

== system LDW_mask/LDW Model/Subsystem1/Departure Warning/Depature detection/subsystem ==
  note: Normal Driving
  note: Meaning of the message: 0 = Right lane departure, 1 = Normal driving, 2 = Left lane departure
  inMsg : Inport
  Bias : Bias  Bias=1
  Combine Left Right Departure : MATLAB Function  TreatAsAtomicUnit=on
  Counter2 : dspswit3/Counter  Direction=Up  CountEvent=Non-zero sample  CounterSize=16 bits  MaxCount=255  InitialCount=0  Output=Count  HitValue=32  ResetInput=on  SamplesPerFrame=1  Ts=1  CntDtype=int32  HitDtype=Logical
  Delay : dspsigops/Delay  dly_unit=Samples  delay=1  ic_detail=off  dif_ic_for_ch=off  dif_ic_for_dly=off  ic=int8(-1)  reset_popup=None
  Detect Change1 : simulink/Logic and Bit Operations/Detect Change  vinit=0  OutDataTypeStr=uint8
  outMsg : Outport
  wires:
  inMsg/1 -> Combine Left Right Departure/1(curMsg), Detect Change1/1, Bias/1
  Delay/1 -> Combine Left Right Departure/2(prevMsg)
  Combine Left Right Departure/1(outMsg) -> outMsg/1, Delay/1
  Detect Change1/1 -> Counter2/2
  Bias/1 -> Counter2/1
  Counter2/1 -> Combine Left Right Departure/3(numNormalDrivenFrames)

== system LDW_mask/LDW Model/Subsystem1/Departure Warning/Depature detection1/subsystem ==
  note: Normal Driving
  note: Meaning of the message: 0 = Right lane departure, 1 = Normal driving, 2 = Left lane departure
  inMsg : Inport
  Bias : Bias  Bias=1
  Combine Left Right Departure : MATLAB Function  TreatAsAtomicUnit=on
  Counter2 : dspswit3/Counter  Direction=Up  CountEvent=Non-zero sample  CounterSize=16 bits  MaxCount=255  InitialCount=0  Output=Count  HitValue=32  ResetInput=on  SamplesPerFrame=1  Ts=1  CntDtype=int32  HitDtype=Logical
  Delay : dspsigops/Delay  dly_unit=Samples  delay=1  ic_detail=off  dif_ic_for_ch=off  dif_ic_for_dly=off  ic=int8(-1)  reset_popup=None
  Detect Change1 : simulink/Logic and Bit Operations/Detect Change  vinit=0  OutDataTypeStr=uint8
  outMsg : Outport
  wires:
  inMsg/1 -> Combine Left Right Departure/1(curMsg), Detect Change1/1, Bias/1
  Delay/1 -> Combine Left Right Departure/2(prevMsg)
  Combine Left Right Departure/1(outMsg) -> outMsg/1, Delay/1
  Detect Change1/1 -> Counter2/2
  Bias/1 -> Counter2/1
  Counter2/1 -> Combine Left Right Departure/3(numNormalDrivenFrames)

== system LDW_mask/LDW Model/Subsystem1/Departure Warning/Find the left and  right lanes from the depository/Search for the left and right lanes ==
  note: Find the line which intersects with the image bottom boundary to the left (right) and which is the closest to the image bottom boundary center.
  Enable : Inport
  Pts : Inport  Port=2
  Half_width : Inport  Port=3
  Dis_inf : Inport  Port=4
  Abs : Abs
  Add2 : Sum  Inputs=+-
  Data Type  Conversion1 : DataTypeConversion  OutDataTypeStr=int32  SaturateOnIntegerOverflow=on  RndMeth=Zero
  Data Type  Conversion2 : DataTypeConversion  OutDataTypeStr=int32  SaturateOnIntegerOverflow=on  RndMeth=Zero
  Intersection with  bottom image boundary{,1..3} (4 alike) : Switch  Criteria=u2 ~= 0  ZeroCross=off
  Left lane? : simulink/Logic and Bit Operations/Compare To Zero  relop=>=  OutDataTypeStr=boolean  ZeroCross=off
  Logical Operator : Logic  AllPortsSameDT=off  OutDataTypeStr=boolean
  Min_left_dis : UnitDelay  X0=single(intmax('int16'))  SampleTime=-1
  Min_left_pts : UnitDelay  X0=[0; 0; 0; 0]  SampleTime=-1
  Relational Operator : RelationalOperator  OutDataTypeStr=boolean  ZeroCross=off
  Relational Operator1 : RelationalOperator  Operator=<=  OutDataTypeStr=boolean
  c1 : Selector  InputPortWidth=4  IndexOptions=Index vector (dialog)  Indices=2  OutputSizes=1
  c2 : Selector  InputPortWidth=4  IndexOptions=Index vector (dialog)  Indices=4  OutputSizes=1
  r1 : Selector  InputPortWidth=4  IndexOptions=Index vector (dialog)  Indices=1  OutputSizes=1
  r2 : Selector  InputPortWidth=4  IndexOptions=Index vector (dialog)  Indices=3  OutputSizes=1
  Left_pts : Outport
  Left_dis : Outport  Port=2
  wires:
  r1/1 -> Relational Operator/1
  r2/1 -> Relational Operator/2
  Relational Operator/1 -> Intersection with  bottom image boundary/2
  c1/1 -> Intersection with  bottom image boundary/1
  c2/1 -> Intersection with  bottom image boundary/3
  Intersection with  bottom image boundary/1 -> Add2/2
  Add2/1 -> Left lane?/1, Abs/1
  Min_left_dis/1 -> Intersection with  bottom image boundary2/1, Relational Operator1/1
  Relational Operator1/1 -> Intersection with  bottom image boundary2/2, Intersection with  bottom image boundary3/2
  Abs/1 -> Intersection with  bottom image boundary1/1
  Dis_inf/1 -> Intersection with  bottom image boundary1/3
  Intersection with  bottom image boundary1/1 -> Relational Operator1/2, Intersection with  bottom image boundary2/3
  Intersection with  bottom image boundary2/1 -> Data Type  Conversion2/1, Left_dis/1
  Min_left_pts/1 -> Intersection with  bottom image boundary3/1
  Intersection with  bottom image boundary3/1 -> Data Type  Conversion1/1, Left_pts/1
  Pts/1 -> r2/1, c2/1, r1/1, c1/1, Intersection with  bottom image boundary3/3
  Half_width/1 -> Add2/1
  Logical Operator/1 -> Intersection with  bottom image boundary1/2
  Left lane?/1 -> Logical Operator/1
  Enable/1 -> Logical Operator/2
  Data Type  Conversion1/1 -> Min_left_pts/1
  Data Type  Conversion2/1 -> Min_left_dis/1

== system LDW_mask/LDW Model/Subsystem1/Departure Warning/Find the left and  right lanes from the depository1/Search for the left and right lanes ==
  note: Find the line which intersects with the image bottom boundary to the left (right) and which is the closest to the image bottom boundary center.
  Enable : Inport
  Pts : Inport  Port=2
  Half_width : Inport  Port=3
  Dis_inf : Inport  Port=4
  Abs : Abs
  Add2 : Sum  Inputs=+-
  Data Type  Conversion1 : DataTypeConversion  OutDataTypeStr=int32  SaturateOnIntegerOverflow=on  RndMeth=Zero
  Data Type  Conversion2 : DataTypeConversion  OutDataTypeStr=int32  SaturateOnIntegerOverflow=on  RndMeth=Zero
  Intersection with  bottom image boundary{,1..3} (4 alike) : Switch  Criteria=u2 ~= 0  ZeroCross=off
  Left lane? : simulink/Logic and Bit Operations/Compare To Zero  relop=>=  OutDataTypeStr=boolean  ZeroCross=off
  Logical Operator : Logic  AllPortsSameDT=off  OutDataTypeStr=boolean
  Min_left_dis : UnitDelay  X0=single(intmax('int16'))  SampleTime=-1
  Min_left_pts : UnitDelay  X0=[0; 0; 0; 0]  SampleTime=-1
  Relational Operator : RelationalOperator  OutDataTypeStr=boolean  ZeroCross=off
  Relational Operator1 : RelationalOperator  Operator=<=  OutDataTypeStr=boolean
  c1 : Selector  InputPortWidth=4  IndexOptions=Index vector (dialog)  Indices=2  OutputSizes=1
  c2 : Selector  InputPortWidth=4  IndexOptions=Index vector (dialog)  Indices=4  OutputSizes=1
  r1 : Selector  InputPortWidth=4  IndexOptions=Index vector (dialog)  Indices=1  OutputSizes=1
  r2 : Selector  InputPortWidth=4  IndexOptions=Index vector (dialog)  Indices=3  OutputSizes=1
  Left_pts : Outport
  Left_dis : Outport  Port=2
  wires:
  Data Type  Conversion2/1 -> Min_left_dis/1
  Data Type  Conversion1/1 -> Min_left_pts/1
  Enable/1 -> Logical Operator/2
  Left lane?/1 -> Logical Operator/1
  Logical Operator/1 -> Intersection with  bottom image boundary1/2
  Half_width/1 -> Add2/1
  Pts/1 -> c1/1, Intersection with  bottom image boundary3/3, r1/1, c2/1, r2/1
  Intersection with  bottom image boundary3/1 -> Data Type  Conversion1/1, Left_pts/1
  Min_left_pts/1 -> Intersection with  bottom image boundary3/1
  Intersection with  bottom image boundary2/1 -> Data Type  Conversion2/1, Left_dis/1
  Intersection with  bottom image boundary1/1 -> Intersection with  bottom image boundary2/3, Relational Operator1/2
  Dis_inf/1 -> Intersection with  bottom image boundary1/3
  Abs/1 -> Intersection with  bottom image boundary1/1
  Relational Operator1/1 -> Intersection with  bottom image boundary3/2, Intersection with  bottom image boundary2/2
  Min_left_dis/1 -> Relational Operator1/1, Intersection with  bottom image boundary2/1
  Add2/1 -> Abs/1, Left lane?/1
  Intersection with  bottom image boundary/1 -> Add2/2
  c2/1 -> Intersection with  bottom image boundary/3
  c1/1 -> Intersection with  bottom image boundary/1
  Relational Operator/1 -> Intersection with  bottom image boundary/2
  r2/1 -> Relational Operator/2
  r1/1 -> Relational Operator/1

== system LDW_mask/LDW Model/Subsystem1/Lane Detection/Peak detection/Enable signal generator ==
  Num : Inport
  Assignment : Assignment  NumberOfDimensions=2  IndexOptions=Assign all,Index vector (port)  Indices=-1,1  OutputSizes=1,1
  Constant : Constant  Value=zeros(1, expLaneNum)  VectorParams1D=off  OutDataTypeStr=boolean
  Constant1 : Constant  VectorParams1D=off  OutDataTypeStr=boolean
  For Iterator : ForIterator  ResetStates=reset  IterationSource=external
  Enable : Outport
  wires:
  For Iterator/1 -> Assignment/3
  Constant1/1 -> Assignment/2
  Assignment/1 -> Enable/1
  Constant/1 -> Assignment/1
  Num/1 -> For Iterator/1

== system LDW_mask/LDW Model/Subsystem1/Lane Detection/Peak detection1/Enable signal generator ==
  Num : Inport
  Assignment : Assignment  NumberOfDimensions=2  IndexOptions=Assign all,Index vector (port)  Indices=-1,1  OutputSizes=1,1
  Constant : Constant  Value=zeros(1, expLaneNum)  VectorParams1D=off  OutDataTypeStr=boolean
  Constant1 : Constant  VectorParams1D=off  OutDataTypeStr=boolean
  For Iterator : ForIterator  ResetStates=reset  IterationSource=external
  Enable : Outport
  wires:
  Num/1 -> For Iterator/1
  Constant/1 -> Assignment/1
  Assignment/1 -> Enable/1
  Constant1/1 -> Assignment/2
  For Iterator/1 -> Assignment/3

== system LDW_mask/LDW Model/Subsystem1/Lane Tracking/Matching/Calculate the distances between  the lines found in the current  frame and those in the respository ==
  Count : Inport
  Rep_ref : Inport  Port=2
  Line : Inport  Port=3
  Enable : Inport  Port=4
  For Iterator : ForIterator  ResetStates=reset  IterationLimit=maxLaneNum
  "Select a line from the repository; if it is valid (Count > 0),  Calculate its distance to the input lines." : Subsystem
  Selector1 : Selector  NumberOfDimensions=2  InputPortWidth=3  IndexOptions=Select all,Index vector (port)  Indices=-1,-1  OutputSizes=1
  Dis : Outport
  wires:
  Enable/1 -> "Select a line from the repository; if it is valid (Count > 0),  Calculate its distance to the input lines."/4(Enable)
  For Iterator/1 -> Selector1/2, "Select a line from the repository; if it is valid (Count > 0),  Calculate its distance to the input lines."/1(Idx)
  "Select a line from the repository; if it is valid (Count > 0),  Calculate its distance to the input lines."/1(Dis) -> Dis/1
  Rep_ref/1 -> "Select a line from the repository; if it is valid (Count > 0),  Calculate its distance to the input lines."/2(Rep_ref)
  Line/1 -> "Select a line from the repository; if it is valid (Count > 0),  Calculate its distance to the input lines."/3(Line)
  Count/1 -> Selector1/1
  Selector1/1 -> "Select a line from the repository; if it is valid (Count > 0),  Calculate its distance to the input lines."/Enable
